simulink model "Project3_Trial"  (R2014a)
settings: Solver=ode45  StartTime=0.0  StopTime=Sim_Time  MaxStep=0.01  RelTol=1e-3
values from neighbouring files (symbols this model uses):
  b = 1    [Project3_Run_Trial.m]
  F = 1    [Project3_Run_Trial.m]
  k = 20    [Project3_Run_Trial.m]
  M = 1    [Project3_Run_Trial.m]
settings Model: Creator=dzr3qn  LastModifiedBy=dzr3qn

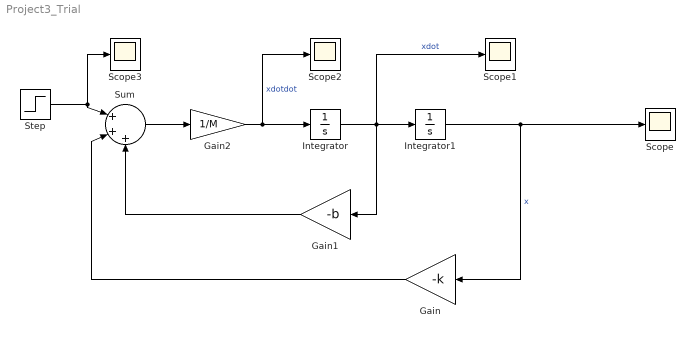
== system Project3_Trial ==
  Gain : Gain  Gain=-k
  Gain1 : Gain  Gain=-b
  Gain2 : Gain  Gain=1/M
  Integrator : Integrator
  Integrator1 : Integrator
  Scope{,1..3} (4 alike) : Scope
      Scope settings: MaxDataPoints=50000
      Scope2 settings: SaveName=ScopeData2
      Scope3 settings: SaveName=ScopeData3
  Step : Step  After=F  SampleTime=0
  Sum : Sum  Inputs=|+++
  wires:
  Gain2/1 -> Scope2/1, Integrator/1  "xdotdot"
  Integrator/1 -> Scope1/1, Gain1/1, Integrator1/1  "xdot"
  Integrator1/1 -> Scope/1, Gain/1  "x"
  Step/1 -> Sum/1, Scope3/1
  Gain1/1 -> Sum/3
  Gain/1 -> Sum/2
  Sum/1 -> Gain2/1
